simulink model "EngineInertia"  (R2025b)
settings: Solver=FixedStepAuto  StartTime=0.0  StopTime=10.0  RelTol=1e-3
undefined symbols (not defined in the file): initial_omega_e, theta_e
settings Model: Creator=rapha  LastModifiedBy=khanh

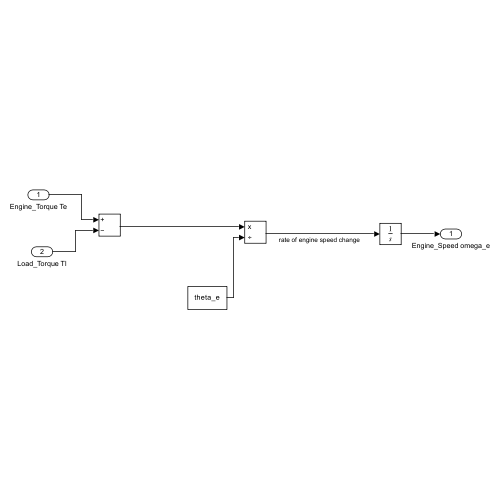
[thumbnail: Simulink's stored preview of the top-level diagram]
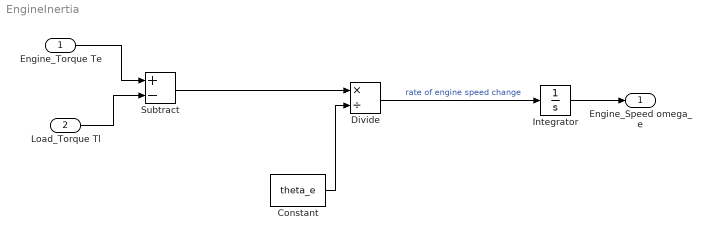
== system EngineInertia ==
  Engine_Torque Te : Inport
  Load_Torque Tl : Inport  Port=2
  Constant : Constant  Value=theta_e
  Divide : Product  Inputs=*/
  Integrator : Integrator  InitialCondition=initial_omega_e
  Subtract : Sum  Inputs=+-
  Engine_Speed omega_e : Outport
  wires:
  Engine_Torque Te/1 -> Subtract/1
  Load_Torque Tl/1 -> Subtract/2
  Subtract/1 -> Divide/1
  Constant/1 -> Divide/2
  Divide/1 -> Integrator/1  "rate of engine speed change"
  Integrator/1 -> Engine_Speed omega_e/1
